simulink model "ACCSim1"  (R2019b)
settings: Solver=FixedStepAuto  StartTime=0.0  StopTime=T  RelTol=1e-3
values from neighbouring files (symbols this model uses):
  t_gap = 1.4    [ACCSim.mat]
  Ts = 0.1    [ACCSim.mat]
  v0_ego = 20    [ACCSim.mat]
  v0_lead = 25    [ACCSim.mat]
  v_set = 30    [ACCSim.mat]
  x0_ego = 10    [ACCSim.mat]
  x0_lead = 50    [ACCSim.mat]
libraries: sim3dautolib x2, mpcadaslib x1, sim3dlib x1
settings Model: Creator=The MathWorks, Inc.  LastModifiedBy=Raymo
settings DataIOCC: ReturnWorkspaceOutputs=off
settings DebuggingCC: ArithmeticOperatorsInVariantConditions=warning
settings SFSimCC: SimUseLocalCustomCode=off  CustomCodeUndefinedFunction=UseInterfaceOnly
settings RTWCC: RTWUseLocalCustomCode=off
settings CodeAppCC: StateflowObjectComments=on

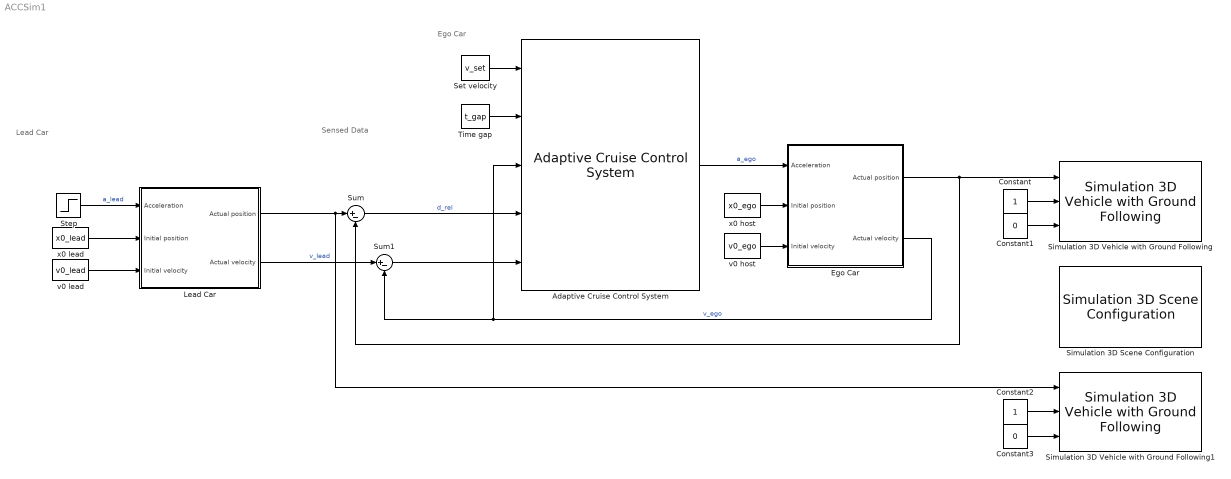
== system ACCSim1 ==
  note: Sensed Data
  note: Lead Car
  note: Ego Car
  Adaptive Cruise Control System : mpcadaslib/Adaptive Cruise Control System  EgoModel=tf(1,[0.5,1,0])  InitialEgoVelocity=20  DefaultSpacing=10  MaxVelocity=50  MinAcceleration=-3  amin_ext=off  MaxAcceleration=2  amax_ext=off  Ts=0.1  PredictionHorizon=30  ControllerBehavior=0.5  suboptimal=off  maxiter=10  datatypeopt=double  optmode=off  trackmode=off
      settings: SourceProductName=Model Predictive Control Toolbox
  Constant : Constant
  Constant1 : Constant  Value=0
  Constant2 : Constant
  Constant3 : Constant  Value=0
  Ego Car : Subsystem
  Lead Car : Subsystem
  Set velocity : Constant  Value=v_set  SampleTime=Ts
  Simulation 3D Scene Configuration : sim3dlib/Simulation 3D Scene Configuration  Priority=0  SceneDesc=Straight road  vehTagList={'Ego';'Scene Origin'}  vehTag=Ego  OpVisEn=off  Ts=1/60  ProjectFormat=Executable  ProjectName=VehicleSimulation.exe  sensorTag=MainCamera1  sensorId=1  sensorName=MainCamera1  mountLoc=Origin  offsetFlag=off  tmountOffset=[0, 0, 0]  rmountOffset=[0, 0, 0]  HorizontalResolution=1280  VerticalResolution=720  HorizontalFOV=60  mountPoint=[0 0 0]  mountOrientation=[0 0 0]  aMode=3  ID=1
      settings: SourceProductName=Automated Driving Toolbox  SourceProductBaseCode=DR
  Simulation 3D Vehicle with Ground Following : sim3dautolib/Simulation 3D Vehicle with Ground Following  Priority=-1  PassVehMesh=Muscle car  VehColor=Yellow  InitialPos=[x0_ego, 2, 0]  InitialRot=[0, 0, 0]  ActorName=Ego  SampleTime=-1  ActorType=SimulinkVehicle  ID=C  aMode=3  ActorTag=Ego  CoordinateScheme=ISO  TransformOutportEnabled=off
      settings: SourceProductName=Automated Driving Toolbox  SourceProductBaseCode=DR
  Simulation 3D Vehicle with Ground Following1 : sim3dautolib/Simulation 3D Vehicle with Ground Following  Priority=-1  PassVehMesh=Hatchback  VehColor=Blue  InitialPos=[x0_lead, 1, 0]  InitialRot=[0, 0, 0]  ActorName=Lead  SampleTime=-1  ActorType=SimulinkVehicle  ID=C  aMode=3  ActorTag=Lead  CoordinateScheme=ISO  TransformOutportEnabled=off
      settings: SourceProductName=Automated Driving Toolbox  SourceProductBaseCode=DR
  Step : Step  Time=5  After=-2  SampleTime=0
  Sum : Sum  Inputs=|+-
  Sum1 : Sum  Inputs=|+-
  Time gap : Constant  Value=t_gap  SampleTime=Ts
  v0 host : Constant  Value=v0_ego  SampleTime=Ts
  v0 lead : Constant  Value=v0_lead  SampleTime=Ts
  x0 host : Constant  Value=x0_ego  SampleTime=Ts
  x0 lead : Constant  Value=x0_lead  SampleTime=Ts
  wires:
  x0 lead/1 -> Lead Car/2(Initial position)
  v0 lead/1 -> Lead Car/3(Initial velocity)
  x0 host/1 -> Ego Car/2(Initial position)
  Ego Car/1(Actual position) -> Simulation 3D Vehicle with Ground Following/1, Sum/2
  Ego Car/2(Actual velocity) -> Adaptive Cruise Control System/3, Sum1/2  "v_ego"
  v0 host/1 -> Ego Car/3(Initial velocity)
  Set velocity/1 -> Adaptive Cruise Control System/1
  Adaptive Cruise Control System/1 -> Ego Car/1(Acceleration)  "a_ego"
  Lead Car/1(Actual position) -> Simulation 3D Vehicle with Ground Following1/1, Sum/1
  Sum1/1 -> Adaptive Cruise Control System/5
  Time gap/1 -> Adaptive Cruise Control System/2
  Step/1 -> Lead Car/1(Acceleration)  "a_lead"
  Lead Car/2(Actual velocity) -> Sum1/1  "v_lead"
  Sum/1 -> Adaptive Cruise Control System/4  "d_rel"
  Constant/1 -> Simulation 3D Vehicle with Ground Following/2
  Constant1/1 -> Simulation 3D Vehicle with Ground Following/3
  Constant2/1 -> Simulation 3D Vehicle with Ground Following1/2
  Constant3/1 -> Simulation 3D Vehicle with Ground Following1/3

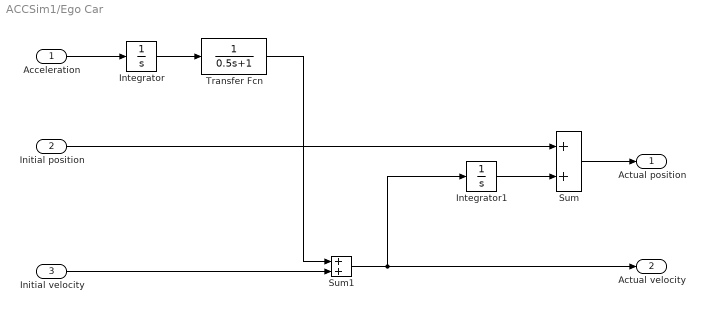
== system ACCSim1/Ego Car ==
  Acceleration : Inport
  Initial position : Inport  Port=2
  Initial velocity : Inport  Port=3
  Integrator : Integrator
  Integrator1 : Integrator
  Sum : Sum
  Sum1 : Sum
  Transfer Fcn : TransferFcn  Denominator=[0.5 1]
  Actual position : Outport  VectorParamsAs1DForOutWhenUnconnected=off
  Actual velocity : Outport  Port=2  VectorParamsAs1DForOutWhenUnconnected=off
  wires:
  Sum1/1 -> Integrator1/1, Actual velocity/1
  Initial velocity/1 -> Sum1/2
  Sum/1 -> Actual position/1
  Transfer Fcn/1 -> Sum1/1
  Integrator/1 -> Transfer Fcn/1
  Acceleration/1 -> Integrator/1
  Initial position/1 -> Sum/1
  Integrator1/1 -> Sum/2

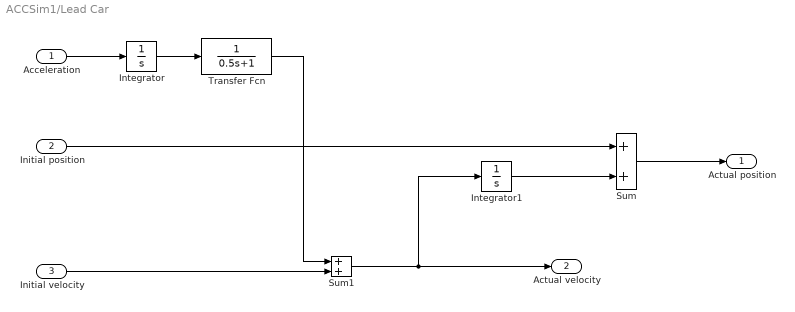
== system ACCSim1/Lead Car ==
  Acceleration : Inport
  Initial position : Inport  Port=2
  Initial velocity : Inport  Port=3
  Integrator : Integrator
  Integrator1 : Integrator
  Sum : Sum
  Sum1 : Sum
  Transfer Fcn : TransferFcn  Denominator=[0.5 1]
  Actual position : Outport  VectorParamsAs1DForOutWhenUnconnected=off
  Actual velocity : Outport  Port=2  VectorParamsAs1DForOutWhenUnconnected=off
  wires:
  Transfer Fcn/1 -> Sum1/1
  Initial velocity/1 -> Sum1/2
  Sum/1 -> Actual position/1
  Integrator/1 -> Transfer Fcn/1
  Sum1/1 -> Integrator1/1, Actual velocity/1
  Acceleration/1 -> Integrator/1
  Initial position/1 -> Sum/1
  Integrator1/1 -> Sum/2
